simulink model "model_task_par_block1"  (R2025b)
settings: Solver=FixedStepDiscrete  StartTime=0.0  StopTime=15.0  FixedStep=0.1  RelTol=1e-3
settings Model: SimulationMode=rapid-accelerator  ExplicitPartitioning=on  Creator=jgillis  LastModifiedBy=jgillis
settings RTWCC: GenCodeOnly=on
settings CodeAppCC: MaxIdLength=1000.0
settings GRTTargetCC: MatFileLogging=off

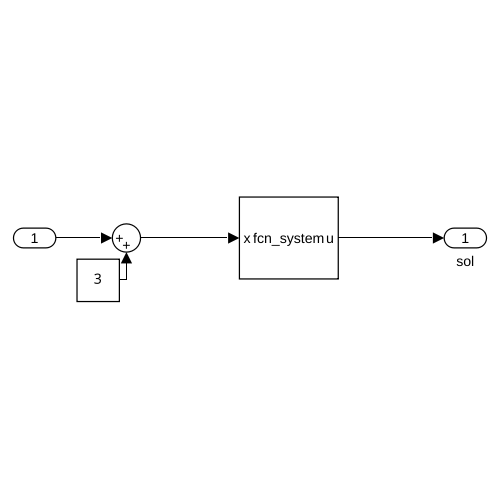
[thumbnail: Simulink's stored preview of the top-level diagram]
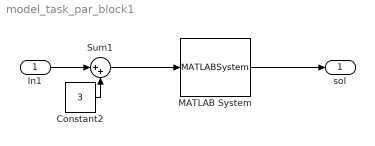
== system model_task_par_block1 ==
  In1 : Inport
  Constant2 : Constant  Value=3
  MATLAB System : MATLABSystem  System=fcn_system  SimulateUsing=Code generation
      mask Type: fcn_system
  Sum1 : Sum  Inputs=|++
  sol : Outport  VectorParamsAs1DForOutWhenUnconnected=off
  wires:
  Sum1/1 -> MATLAB System/1
  Constant2/1 -> Sum1/2
  In1/1 -> Sum1/1
  MATLAB System/1 -> sol/1
